simulink model "PubIfCommonEHRV2_MDL"  (R2020b)
settings: Solver=FixedStepAuto  StartTime=0.0  StopTime=Inf  RelTol=1e-3
PostLoadFcn:
  | if any(exist('dsrtsu_mdlpostloadfcn', 'file') ~= 0), dsrtsu_mdlpostloadfcn('Execute', bdroot); end
InitFcn:
  | , if any(exist('dsmpb_private', 'file') ~= 0), dsmpb_private('dsmpb_mdlclblib', 'Init', bdroot); end,
undefined symbols (not defined in the file): CAMERA_STATE_INITIAL, CAMERA_STATE_NORMAL, CURVATURE_UNKNOWN, DISTANCE_UNKONWN, DRIVING_ON_HIGHWAY_YES, EHR_CYCLE, FORWARD_LOOKING_DISTANCE_LIMIT, IFC_HUT_INTERFACE_NO_RESPONSE, IFC_HUT_INTERFACE_RESPONSE, MAP_DATA_VALID_VALID, MSG_TYPE_PROFILE_LONG, MSG_TYPE_PROFILE_SHORT, MSG_TYPE_SEGMENT, MSG_TYPE_STUB, OFFSET_INVALID, OFFSET_MAX, P_EHRV2_dCurvatureFar, P_EHRV2_dCurvatureMatrix, P_EHRV2_dSlopeFar, P_EHRV2_dSlopeMatrix, P_EHRV2_dVehForwardLooking, P_EHRV2_dVehRearLooking, P_EHRV2_tIFCHUTNoResponseOfForecastTreeReset, P_EHRV2_tIFCHUTNoResponseOfTimeout, P_EHRV2_tIFCHUTResponseTimeout, PROFILE_SHORT_NO_OTHER_VALUE, PROFILE_SHORT_TYPE_CURVATURE, PROFILE_SHORT_TYPE_SLOPE, REAR_LOOKING_DISTANCE_LIMIT, SLOPE_UNKNOWN, STUB_CMPLX_INSCT, STUB_FORM_OF_WAY_HIGH_RING_ROAD, STUB_FORM_OF_WAY_NORMAL_RING_ROAD
libraries: simulink x5
(part 1 of 4)
PreSaveFcn:
  | , if any(exist('dsmpb_private', 'file') ~= 0), dsmpb_private('dsmpb_mdlclblib', 'PreSave', bdroot); end,
CloseFcn:
  | , if any(exist('dsmpb_private', 'file') ~= 0), dsmpb_private('dsmpb_mdlclblib', 'Close', bdroot); end,
settings Model: DataDictionary=HWA_DDs.sldd  RTICANMMDATA=struct('GeneralSetupData',struct('modelroot','C:\Users\GW00133806\Desktop\ADAS_Store\Adas\EHR','generalsettings',struct('filesettings',struct('destfolder',struct('Name','RTICANMM_FILES','Check',1),'buildfolder',struct('Name','.','Check',1),'AbsDestfolder',struct('Name','C:\Users\GW00133806\Desktop\ADAS_Store\Adas\EHR\RTICANMM_FILES'),'AbsBuildfolder',struct('Name','C:\Users\GW00133806\Desktop\ADAS_Store\Adas\EHR'))),'options',struct('addpaths',1,'rmpaths',1,'addtrcexclusion',false,'cannavigator',struct('checkmonitoring',0),'show_usrtrc',0,'use_usrtrc',0),'advanced',struct('options',ones(1,100)),'MPSetup',{{}},'RTI',struct('Type','DSRT','Ver','4.2','Date','02-Nov-2019'),'modelname','PubIfCommonEHRV2_MDL','block','PubIfCommonEHRV2_MDL'))  DSRTSU_INTERNAL_RTIFPGA=150  Creator=GW00180895  LastModifiedBy=GW00133806
settings OptimizationCC: BlockReduction=off  ConditionallyExecuteInputs=off  OptimizeBlockIOStorage=off  BufferReuse=off  GlobalBufferReuse=off  ExpressionFolding=off  LocalBlockOutputs=off  OptimizeDataStoreBuffers=off  BusAssignmentInplaceUpdate=off
settings DebuggingCC: TasksWithSamePriorityMsg=none
settings HardwareCC: ProdBitPerPointer=32  ProdBitPerSizeT=32  ProdBitPerPtrDiffT=32  ProdLargestAtomicInteger=Integer  ProdWordSize=32  ProdHWDeviceType=Custom Processor->Custom
settings ModelReferenceCC: UpdateModelReferenceTargets=AssumeUpToDate  EnableParallelModelReferenceBuilds=on  ModelReferenceNumInstancesAllowed=Single
settings SFSimCC: MATLABDynamicMemAlloc=off
settings RTWCC: Description=dSPACE Run-Time Target (for VEOS on Windows and ConfigurationDesk)  SystemTargetFile=dsrt.tlc  GenCodeOnly=on  MakeCommand=make_dsrt  TemplateMakefile=dsrt_default_tmf  RTWVerbose=off
settings CodeAppCC: MaxIdLength=128
settings STFCustomTargetCC: TargetLangStandard=C99 (ISO)  ParMdlRefBuildCompliant=on  ConcurrentExecutionCompliant=off  CPPClassGenCompliant=off  GRTInterface=off  SystemTargetFile=dsrt.tlc
settings GRTTargetCC: CompOptLevelCompliant=off  ConcurrentExecutionCompliant=off  CombineOutputUpdateFcns=off  MatFileLogging=off  CPPClassGenCompliant=off  UseToolchainInfoCompliant=off

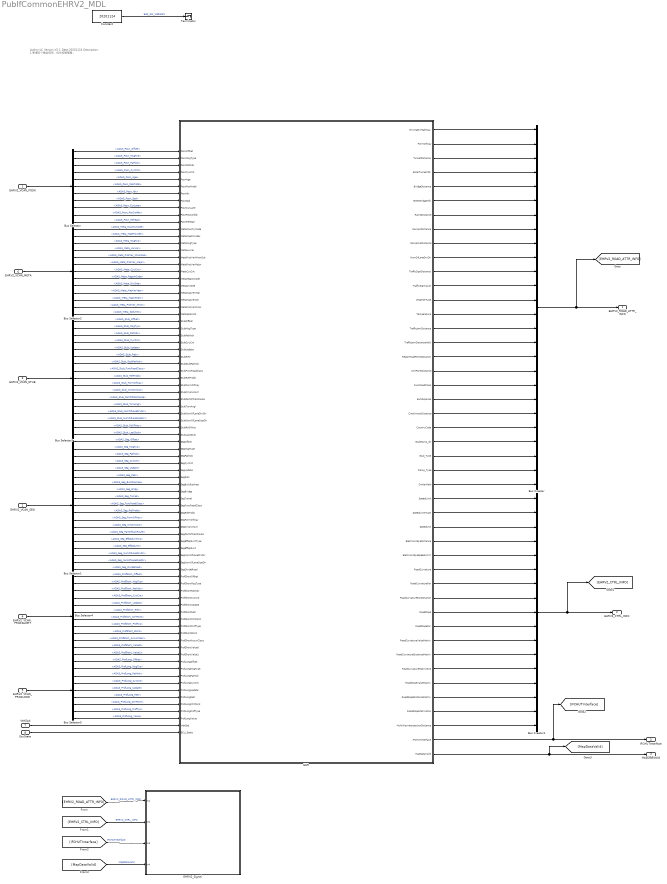
== system PubIfCommonEHRV2_MDL ==
  note: Author:LC
      | Version:V2.1
      | Data:20201124
      | Description:
      | 1.新增五个输出信号，优化控制策略；
  EHRV2_VCAN_POSN : Inport  OutDataTypeStr=Bus: EHRV2_VCAN_POSN_BUS  PortDimensions=1  BusOutputAsStruct=on
  EHRV2_VCAN_SEG : Inport  Port=2  OutDataTypeStr=Bus: EHRV2_VCAN_SEG_BUS  PortDimensions=1  BusOutputAsStruct=on
  EHRV2_VCAN_STUB : Inport  Port=3  OutDataTypeStr=Bus: EHRV2_VCAN_STUB_BUS  PortDimensions=1  BusOutputAsStruct=on
  EHRV2_VCAN_PROFSHORT : Inport  Port=4  OutDataTypeStr=Bus: EHRV2_VCAN_PROFSHORT_BUS  PortDimensions=1  BusOutputAsStruct=on
  EHRV2_VCAN_PROFLONG : Inport  Port=5  OutDataTypeStr=Bus: EHRV2_VCAN_PROFLONG_BUS  PortDimensions=1  BusOutputAsStruct=on
  EHRV2_VCAN_META : Inport  Port=6  OutDataTypeStr=Bus: EHRV2_VCAN_META_BUS  PortDimensions=1  BusOutputAsStruct=on
  VehSpd : Inport  Port=7  OutDataTypeStr=single  PortDimensions=1  BusOutputAsStruct=on
  EcuState : Inport  Port=8  OutDataTypeStr=uint8  PortDimensions=1  BusOutputAsStruct=on
  Bus Creator : BusCreator  Inputs=26
  Bus Creator1 : BusCreator  Inputs=17
  Bus Selector : BusSelector  OutputSignals=ADAS_Posn_Offset,ADAS_Posn_MsgTye,ADAS_Posn_Pathldx,ADAS_Posn_CycCnt,ADAS_Posn_Age,ADAS_Posn_PosProbb,ADAS_Posn_Idx,ADAS_Posn_Spd,ADAS_Posn_CurLane,ADAS_Posn_PosConfdc,ADAS_Posn_Rehead
  Bus Selector1 : BusSelector  OutputSignals=ADAS_Seg_Offset,ADAS_Seg_MsgTyp,ADAS_Seg_PathIdx,ADAS_Seg_CycCnt,ADAS_Seg_Update,ADAS_Seg_Retr,ADAS_Seg_BuildUpArea,ADAS_Seg_Brdg,ADAS_Seg_Tunnel,ADAS_Seg_FuncRoadClass,ADAS_Seg_RelProbb,ADAS_Seg_FormOfWay,ADAS_Seg_CmplxInsct,ADAS_Seg_PartOfCalcRoute,ADAS_Seg_EffSpdLmtTyp,ADAS_Seg_EffSpdLmt,ADAS_Seg_NumOfLaneDrvDir,ADAS_Seg_NumOfLaneOppDir,ADAS_Seg_DivideRoad
  Bus Selector2 : BusSelector  OutputSignals=ADAS_Meta_CountryCode,ADAS_Meta_MapProvider,ADAS_Meta_MsgTyp,ADAS_Meta_HwVer,ADAS_Meta_ProtVer_MinorSub,ADAS_Meta_ProtVer_Major,ADAS_Meta_CycCnt,ADAS_Meta_RegionCode,ADAS_Meta_DrvSide,ADAS_Meta_MapVerYear,ADAS_Meta_MapVerQtr,ADAS_Meta_ProtVer_Minor,ADAS_Meta_SpdUnits
  Bus Selector3 : BusSelector  OutputSignals=ADAS_Stub_Offset,ADAS_Stub_MsgTyp,ADAS_Stub_PathIdx,ADAS_Stub_CycCnt,ADAS_Stub_Update,ADAS_Stub_Retr,ADAS_Stub_StubPathIdx,ADAS_Stub_FuncRoadClass,ADAS_Stub_RelProbb,ADAS_Stub_FormOfWay,ADAS_Stub_CmplxInsct,ADAS_Stub_PartOfCalcRoute,ADAS_Stub_TurnAngl,ADAS_Stub_NumOfLaneDrvDir,ADAS_Stub_NumOfLaneOppDir,ADAS_Stub_RtOfWay,ADAS_Stub_LastStub
  Bus Selector4 : BusSelector  OutputSignals=ADAS_ProfShort_Offset,ADAS_ProfShort_MsgTyp,ADAS_ProfShort_PathIdx,ADAS_ProfShort_CycCnt,ADAS_ProfShort_Update,ADAS_ProfShort_Retr,ADAS_ProfShort_CtrlPoint,ADAS_ProfShort_ProfTyp,ADAS_ProfShort_Dist1,ADAS_ProfShort_AccurClass,ADAS_ProfShort_Value0,ADAS_ProfShort_Value1
  Bus Selector5 : BusSelector  OutputSignals=ADAS_ProfLong_Offset,ADAS_ProfLong_MsgTyp,ADAS_ProfLong_PathIdx,ADAS_ProfLong_CycCnt,ADAS_ProfLong_Update,ADAS_ProfLong_Retr,ADAS_ProfLong_CtrlPoint,ADAS_ProfLong_ProfTyp,ADAS_ProfLong_Value
  Constant : Constant  Value=20201124  OutDataTypeStr=uint32
  EHR : Subsystem
  EHRV2_Signal : Subsystem
  Terminator : Terminator
  EHRV2_ROAD_ATTR_INFO : Outport  OutDataTypeStr=Bus: EHRV2_ROAD_ATTR_INFO_BUS  PortDimensions=1  BusOutputAsStruct=on
  EHRV2_CTRL_INFO : Outport  Port=2  OutDataTypeStr=Bus: EHRV2_CTRL_INFO_BUS  PortDimensions=1  BusOutputAsStruct=on
  IFCHUTInterface : Outport  Port=3  OutDataTypeStr=uint8  PortDimensions=1  BusOutputAsStruct=on
  MapDataValid : Outport  Port=4  OutDataTypeStr=uint8  PortDimensions=1  BusOutputAsStruct=on
  wires:
  Bus Selector3/17 -> EHR/41(StubLastStub)  "<ADAS_Stub_LastStub>"
  EHR/25(Ramp_Type) -> Bus Creator/25
  Bus Selector3/16 -> EHR/40(StubRtOfWay)  "<ADAS_Stub_RtOfWay>"
  EHR/32(RoadCurvature) -> Bus Creator1/6
  Bus Selector1/11 -> EHR/52(SegRelProbb)  "<ADAS_Seg_RelProbb>"
  EHRV2_VCAN_SEG/1 -> Bus Selector1/1
  EHR/2(FormOfWay) -> Bus Creator/2
  Bus Selector/1 -> EHR/1(PosnOffset)  "<ADAS_Posn_Offset>"
  EHR/35(RoadSlope) -> Bus Creator1/9
  VehSpd/1 -> EHR/82(VehSpd)
  Bus Selector/4 -> EHR/4(PosnCycCnt)  "<ADAS_Posn_CycCnt>"
  EHRV2_VCAN_META/1 -> Bus Selector2/1
  Constant/1 -> Terminator/1  "EHR_SW_VERSION"
  EHR/11(TrafficSignDistance) -> Bus Creator/11
  EHR/36(RoadSlopeFar) -> Bus Creator1/10
  Bus Selector2/8 -> EHR/19(MetaRegionCode)  "<ADAS_Meta_RegionCode>"
  EHR/24(Stub_Type) -> Bus Creator/24
  EHR/12(TrafficSignValue) -> Bus Creator/12
  Bus Creator1/1 -> [EHRV2_CTRL_INFO], EHRV2_CTRL_INFO/1
  Bus Selector5/8 -> EHR/80(ProfLongProfType)  "<ADAS_ProfLong_ProfTyp>"
  Bus Selector/3 -> EHR/3(PosnPathIdx)  "<ADAS_Posn_Pathldx>"
  Bus Selector3/5 -> EHR/29(StubUpdate)  "<ADAS_Stub_Update>"
  EHR/23(StubRamp_dir) -> Bus Creator/23
  Bus Selector1/10 -> EHR/51(SegFuncRoadClass)  "<ADAS_Seg_FuncRoadClass>"
  Bus Selector4/4 -> EHR/64(ProfShortCycCnt)  "<ADAS_ProfShort_CycCnt>"
  EHR/43(MultiWayIntersectionDistance) -> Bus Creator1/17
  Bus Selector3/14 -> EHR/38(StubNumOfLaneDrvDir)  "<ADAS_Stub_NumOfLaneDrvDir>"
  Bus Selector2/7 -> EHR/18(MetaCycCnt)  "<ADAS_Meta_CycCnt>"
  EHRV2_VCAN_STUB/1 -> Bus Selector3/1
  EHRV2_VCAN_PROFSHORT/1 -> Bus Selector4/1
  EHR/9(RampOutDistance) -> Bus Creator/9
  EHR/39(RoadCurvatureMatrixSize) -> Bus Creator1/13
  EHRV2_VCAN_PROFLONG/1 -> Bus Selector5/1
  EHR/42(RoadSlopeMatrixSize) -> Bus Creator1/16
  EHR/15(TrafficJamDistance) -> Bus Creator/15
  EHR/29(SpeedUnit) -> Bus Creator1/3
  Bus Selector1/17 -> EHR/58(SegNumOfLaneDrvDir)  "<ADAS_Seg_NumOfLaneDrvDir>"
  Bus Selector4/7 -> EHR/67(ProfShortCtrlPoint)  "<ADAS_ProfShort_CtrlPoint>"
  Bus Selector4/10 -> EHR/70(ProfShortAccurClass)  "<ADAS_ProfShort_AccurClass>"
  Bus Selector3/10 -> EHR/34(StubFormOfWay)  "<ADAS_Stub_FormOfWay>"
  Bus Selector3/11 -> EHR/35(StubCmplxInsct)  "<ADAS_Stub_CmplxInsct>"
  Bus Selector2/6 -> EHR/17(MetaProtVerMajor)  "<ADAS_Meta_ProtVer_Major>"
  EHRV2_VCAN_POSN/1 -> Bus Selector/1
  EHR/41(RoadSlopeDistanceMatrix) -> Bus Creator1/15
  Bus Selector5/1 -> EHR/73(ProfLongOffset)  "<ADAS_ProfLong_Offset>"
  EHR/18(CtrlPointDistance) -> Bus Creator/18
  [IFCHUTInterface] -> EHRV2_Signal/3(In3)  "IFCHUTInterface"
  Bus Selector5/3 -> EHR/75(ProfLongPathIdx)  "<ADAS_ProfLong_PathIdx>"
  Bus Creator/1 -> [EHRV2_ROAD_ATTR_INFO], EHRV2_ROAD_ATTR_INFO/1
  EHR/45(MapDataValid) -> [MapDataValid], MapDataValid/1
  Bus Selector4/9 -> EHR/69(ProfShortDist1)  "<ADAS_ProfShort_Dist1>"
  Bus Selector/8 -> EHR/8(PosnSpd)  "<ADAS_Posn_Spd>"
  Bus Selector1/4 -> EHR/45(SegCycCnt)  "<ADAS_Seg_CycCnt>"
  Bus Selector/10 -> EHR/10(PosnPosConfdc)  "<ADAS_Posn_PosConfdc>"
  Bus Selector4/3 -> EHR/63(ProfShortPathIdx)  "<ADAS_ProfShort_PathIdx>"
  Bus Selector5/9 -> EHR/81(ProfLongValue)  "<ADAS_ProfLong_Value>"
  Bus Selector4/1 -> EHR/61(ProfShortOffset)  "<ADAS_ProfShort_Offset>"
  Bus Selector3/3 -> EHR/27(StubPathIdx)  "<ADAS_Stub_PathIdx>"
  Bus Selector5/4 -> EHR/76(ProfLongCycCnt)  "<ADAS_ProfLong_CycCnt>"
  EHR/17(RepairRoadPointDistance) -> Bus Creator/17
  Bus Selector3/13 -> EHR/37(StubTurnAngl)  "<ADAS_Stub_TurnAngl>"
  EHR/34(RoadCurvatureFarDistance) -> Bus Creator1/8
  EHR/8(RampInDistance) -> Bus Creator/8
  Bus Selector4/12 -> EHR/72(ProfShortValue1)  "<ADAS_ProfShort_Value1>"
  EHR/4(EnterTunnelInfo) -> Bus Creator/4
  Bus Selector2/9 -> EHR/20(MetaDrvSide)  "<ADAS_Meta_DrvSide>"
  EHR/26(OnNavPath) -> Bus Creator/26
  EHR/19(FuncRoadClass) -> Bus Creator/19
  Bus Selector5/7 -> EHR/79(ProfLongCtrlPoint)  "<ADAS_ProfLong_CtrlPoint>"
  Bus Selector1/5 -> EHR/46(SegUpdate)  "<ADAS_Seg_Update>"
  EHR/44(IFCHUTInterface) -> IFCHUTInterface/1, [IFCHUTInterface]
  Bus Selector2/11 -> EHR/22(MetaMapVerQtr)  "<ADAS_Meta_MapVerQtr>"
  Bus Selector3/7 -> EHR/31(StubStubPathIdx)  "<ADAS_Stub_StubPathIdx>"
  Bus Selector2/1 -> EHR/12(MetaCountryCode)  "<ADAS_Meta_CountryCode>"
  EHR/7(RampDistance) -> Bus Creator/7
  Bus Selector3/9 -> EHR/33(StubRelProbb)  "<ADAS_Stub_RelProbb>"
  Bus Selector1/3 -> EHR/44(SegPathIdx)  "<ADAS_Seg_PathIdx>"
  EcuState/1 -> EHR/83(ECU_State)
  Bus Selector1/7 -> EHR/48(SegBuildUpArea)  "<ADAS_Seg_BuildUpArea>"
  Bus Selector/6 -> EHR/6(PosnPosProbb)  "<ADAS_Posn_PosProbb>"
  Bus Selector3/8 -> EHR/32(StubFuncRoadClass)  "<ADAS_Stub_FuncRoadClass>"
  [EHRV2_CTRL_INFO] -> EHRV2_Signal/2(In2)  "EHRV2_CTRL_INFO"
  Bus Selector1/2 -> EHR/43(SegMsgType)  "<ADAS_Seg_MsgTyp>"
  Bus Selector2/3 -> EHR/14(MetaMsgType)  "<ADAS_Meta_MsgTyp>"
  Bus Selector2/5 -> EHR/16(MetaProtVerMinorSub)  "<ADAS_Meta_ProtVer_MinorSub>"
  Bus Selector/9 -> EHR/9(PosnCurLane)  "<ADAS_Posn_CurLane>"
  Bus Selector1/13 -> EHR/54(SegCmplxInsct)  "<ADAS_Seg_CmplxInsct>"
  Bus Selector3/15 -> EHR/39(StubNumOfLaneOppDir)  "<ADAS_Stub_NumOfLaneOppDir>"
  Bus Selector4/6 -> EHR/66(ProfShortRetr)  "<ADAS_ProfShort_Retr>"
  Bus Selector3/2 -> EHR/26(StubMsgType)  "<ADAS_Stub_MsgTyp>"
  Bus Selector1/19 -> EHR/60(SegDivideRoad)  "<ADAS_Seg_DivideRoad>"
  Bus Selector1/16 -> EHR/57(SegEffSpdLmt)  "<ADAS_Seg_EffSpdLmt>"
  Bus Selector4/2 -> EHR/62(ProfShortMsgType)  "<ADAS_ProfShort_MsgTyp>"
  EHR/37(RoadCurvatureValueMatrix) -> Bus Creator1/11
  Bus Selector2/10 -> EHR/21(MetaMapVerYear)  "<ADAS_Meta_MapVerYear>"
  Bus Selector2/2 -> EHR/13(MetaMapProvider)  "<ADAS_Meta_MapProvider>"
  Bus Selector/5 -> EHR/5(PosnAge)  "<ADAS_Posn_Age>"
  Bus Selector1/9 -> EHR/50(SegTunnel)  "<ADAS_Seg_Tunnel>"
  Bus Selector3/6 -> EHR/30(StubRetr)  "<ADAS_Stub_Retr>"
  Bus Selector1/8 -> EHR/49(SegBridge)  "<ADAS_Seg_Brdg>"
  Bus Selector/7 -> EHR/7(PosnIdx)  "<ADAS_Posn_Idx>"
  Bus Selector5/6 -> EHR/78(ProfLongRetr)  "<ADAS_ProfLong_Retr>"
  EHR/10(NumOfLaneDrvDir) -> Bus Creator/10
  Bus Selector5/5 -> EHR/77(ProfLongUpdate)  "<ADAS_ProfLong_Update>"
  Bus Selector2/13 -> EHR/24(MetaSpdUnits)  "<ADAS_Meta_SpdUnits>"
  EHR/30(ElectronicEyeDistance) -> Bus Creator1/4
  Bus Selector/11 -> EHR/11(PosnRehead)  "<ADAS_Posn_Rehead>"
  EHR/16(TrafficJamDistanceHold) -> Bus Creator/16
  EHR/31(ElectronicEyeSpeedLimit) -> Bus Creator1/5
  [EHRV2_ROAD_ATTR_INFO] -> EHRV2_Signal/1(In1)  "EHRV2_ROAD_ATTR_INFO"
  EHR/6(EnterBridgeInfo) -> Bus Creator/6
  Bus Selector4/8 -> EHR/68(ProfShortProfType)  "<ADAS_ProfShort_ProfTyp>"
  Bus Selector/2 -> EHR/2(PosnMsgType)  "<ADAS_Posn_MsgTye>"
  EHR/27(SpeedLimit) -> Bus Creator1/1
  EHR/22(CountryCode) -> Bus Creator/22
  Bus Selector3/12 -> EHR/36(StubPartOfCalcRoute)  "<ADAS_Stub_PartOfCalcRoute>"
  Bus Selector2/4 -> EHR/15(MetaHwVer)  "<ADAS_Meta_HwVer>"
  EHR/20(BuildUpArea) -> Bus Creator/20
  EHR/5(BridgeDistance) -> Bus Creator/5
  Bus Selector4/5 -> EHR/65(ProfShortUpdate)  "<ADAS_ProfShort_Update>"
  Bus Selector3/4 -> EHR/28(StubCycCnt)  "<ADAS_Stub_CycCnt>"
  Bus Selector1/14 -> EHR/55(SegPartOfCalcRoute)  "<ADAS_Seg_PartOfCalcRoute>"
  Bus Selector2/12 -> EHR/23(MetaProtVerMinor)  "<ADAS_Meta_ProtVer_Minor>"
  EHR/13(WeatherType) -> Bus Creator/13
  EHR/33(RoadCurvatureFar) -> Bus Creator1/7
  EHR/14(Temperature) -> Bus Creator/14
  Bus Selector4/11 -> EHR/71(ProfShortValue0)  "<ADAS_ProfShort_Value0>"
  Bus Selector1/18 -> EHR/59(SegNumOfLaneOppDir)  "<ADAS_Seg_NumOfLaneOppDir>"
  Bus Selector1/6 -> EHR/47(SegRetr)  "<ADAS_Seg_Retr>"
  EHR/3(TunnelDistance) -> Bus Creator/3
  Bus Selector1/12 -> EHR/53(SegFormOfWay)  "<ADAS_Seg_FormOfWay>"
  Bus Selector5/2 -> EHR/74(ProfLongMsgType)  "<ADAS_ProfLong_MsgTyp>"
  EHR/21(CmplxInsctDistance) -> Bus Creator/21
  [MapDataValid] -> EHRV2_Signal/4(In4)  "MapDataValid"
  Bus Selector1/15 -> EHR/56(SegEffSpdLmtType)  "<ADAS_Seg_EffSpdLmtTyp>"
  Bus Selector3/1 -> EHR/25(StubOffset)  "<ADAS_Stub_Offset>"
  Bus Selector1/1 -> EHR/42(SegOffset)  "<ADAS_Seg_Offset>"
  EHR/28(SpeedLimitType) -> Bus Creator1/2
  EHR/1(DrivingOnHighWay) -> Bus Creator/1
  EHR/40(RoadSlopeValueMatrix) -> Bus Creator1/14
  EHR/38(RoadCurvatureDistanceMatrix) -> Bus Creator1/12

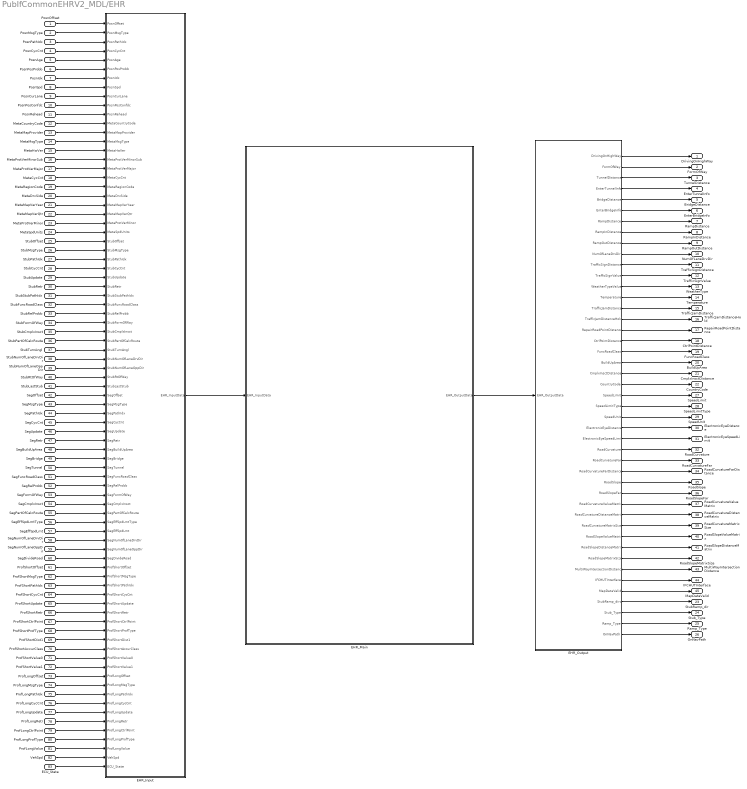
== system PubIfCommonEHRV2_MDL/EHR ==
  PosnOffset : Inport  OutDataTypeStr=uint16  PortDimensions=1
  PosnMsgType : Inport  Port=2  OutDataTypeStr=uint8  PortDimensions=1
  PosnPathIdx : Inport  Port=3  OutDataTypeStr=uint8  PortDimensions=1
  PosnCycCnt : Inport  Port=4  OutDataTypeStr=uint8  PortDimensions=1
  PosnAge : Inport  Port=5  OutDataTypeStr=uint16  PortDimensions=1
  PosnPosProbb : Inport  Port=6  OutDataTypeStr=single  PortDimensions=1
  PosnIdx : Inport  Port=7  OutDataTypeStr=uint8  PortDimensions=1
  PosnSpd : Inport  Port=8  OutDataTypeStr=single  PortDimensions=1
  PosnCurLane : Inport  Port=9  OutDataTypeStr=uint8  PortDimensions=1
  PosnPosConfdc : Inport  Port=10  OutDataTypeStr=uint8  PortDimensions=1
  PosnRehead : Inport  Port=11  OutDataTypeStr=single  PortDimensions=1
  MetaCountryCode : Inport  Port=12  OutDataTypeStr=uint16  PortDimensions=1
  MetaMapProvider : Inport  Port=13  OutDataTypeStr=uint8  PortDimensions=1
  MetaMsgType : Inport  Port=14  OutDataTypeStr=uint8  PortDimensions=1
  MetaHwVer : Inport  Port=15  OutDataTypeStr=uint16  PortDimensions=1
  MetaProtVerMinorSub : Inport  Port=16  OutDataTypeStr=uint8  PortDimensions=1
  MetaProtVerMajor : Inport  Port=17  OutDataTypeStr=uint8  PortDimensions=1
  MetaCycCnt : Inport  Port=18  OutDataTypeStr=uint8  PortDimensions=1
  MetaRegionCode : Inport  Port=19  OutDataTypeStr=uint16  PortDimensions=1
  MetaDrvSide : Inport  Port=20  OutDataTypeStr=boolean  PortDimensions=1
  MetaMapVerYear : Inport  Port=21  OutDataTypeStr=uint8  PortDimensions=1
  MetaMapVerQtr : Inport  Port=22  OutDataTypeStr=uint8  PortDimensions=1
  MetaProtVerMinor : Inport  Port=23  OutDataTypeStr=uint8  PortDimensions=1
  MetaSpdUnits : Inport  Port=24  OutDataTypeStr=boolean  PortDimensions=1
  StubOffset : Inport  Port=25  OutDataTypeStr=uint16  PortDimensions=1
  StubMsgType : Inport  Port=26  OutDataTypeStr=uint8  PortDimensions=1
  StubPathIdx : Inport  Port=27  OutDataTypeStr=uint8  PortDimensions=1
  StubCycCnt : Inport  Port=28  OutDataTypeStr=uint8  PortDimensions=1
  StubUpdate : Inport  Port=29  OutDataTypeStr=boolean  PortDimensions=1
  StubRetr : Inport  Port=30  OutDataTypeStr=boolean  PortDimensions=1
  StubStubPathIdx : Inport  Port=31  OutDataTypeStr=uint8  PortDimensions=1
  StubFuncRoadClass : Inport  Port=32  OutDataTypeStr=uint8  PortDimensions=1
  StubRelProbb : Inport  Port=33  OutDataTypeStr=single  PortDimensions=1
  StubFormOfWay : Inport  Port=34  OutDataTypeStr=uint8  PortDimensions=1
  StubCmplxInsct : Inport  Port=35  OutDataTypeStr=uint8  PortDimensions=1
  StubPartOfCalcRoute : Inport  Port=36  OutDataTypeStr=uint8  PortDimensions=1
  StubTurnAngl : Inport  Port=37  OutDataTypeStr=single  PortDimensions=1
  StubNumOfLaneDrvDir : Inport  Port=38  OutDataTypeStr=uint8  PortDimensions=1
  StubNumOfLaneOppDir : Inport  Port=39  OutDataTypeStr=uint8  PortDimensions=1
  StubRtOfWay : Inport  Port=40  OutDataTypeStr=uint8  PortDimensions=1
  StubLastStub : Inport  Port=41  OutDataTypeStr=boolean  PortDimensions=1
  SegOffset : Inport  Port=42  OutDataTypeStr=uint16  PortDimensions=1
  SegMsgType : Inport  Port=43  OutDataTypeStr=uint8  PortDimensions=1
  SegPathIdx : Inport  Port=44  OutDataTypeStr=uint8  PortDimensions=1
  SegCycCnt : Inport  Port=45  OutDataTypeStr=uint8  PortDimensions=1
  SegUpdate : Inport  Port=46  OutDataTypeStr=boolean  PortDimensions=1
  SegRetr : Inport  Port=47  OutDataTypeStr=boolean  PortDimensions=1
  SegBuildUpArea : Inport  Port=48  OutDataTypeStr=uint8  PortDimensions=1
  SegBridge : Inport  Port=49  OutDataTypeStr=uint8  PortDimensions=1
  SegTunnel : Inport  Port=50  OutDataTypeStr=uint8  PortDimensions=1
  SegFuncRoadClass : Inport  Port=51  OutDataTypeStr=uint8  PortDimensions=1
  SegRelProbb : Inport  Port=52  OutDataTypeStr=single  PortDimensions=1
  SegFormOfWay : Inport  Port=53  OutDataTypeStr=uint8  PortDimensions=1
  SegCmplxInsct : Inport  Port=54  OutDataTypeStr=uint8  PortDimensions=1
  SegPartOfCalcRoute : Inport  Port=55  OutDataTypeStr=uint8  PortDimensions=1
  SegEffSpdLmtType : Inport  Port=56  OutDataTypeStr=uint8  PortDimensions=1
  SegEffSpdLmt : Inport  Port=57  OutDataTypeStr=uint8  PortDimensions=1
  SegNumOfLaneDrvDir : Inport  Port=58  OutDataTypeStr=uint8  PortDimensions=1
  SegNumOfLaneOppDir : Inport  Port=59  OutDataTypeStr=uint8  PortDimensions=1
  SegDivideRoad : Inport  Port=60  OutDataTypeStr=uint8  PortDimensions=1
  ProfShortOffset : Inport  Port=61  OutDataTypeStr=uint16  PortDimensions=1
  ProfShortMsgType : Inport  Port=62  OutDataTypeStr=uint8  PortDimensions=1
  ProfShortPathIdx : Inport  Port=63  OutDataTypeStr=uint8  PortDimensions=1
  ProfShortCycCnt : Inport  Port=64  OutDataTypeStr=uint8  PortDimensions=1
  ProfShortUpdate : Inport  Port=65  OutDataTypeStr=boolean  PortDimensions=1
  ProfShortRetr : Inport  Port=66  OutDataTypeStr=boolean  PortDimensions=1
  ProfShortCtrlPoint : Inport  Port=67  OutDataTypeStr=boolean  PortDimensions=1
  ProfShortProfType : Inport  Port=68  OutDataTypeStr=uint8  PortDimensions=1
  ProfShortDist1 : Inport  Port=69  OutDataTypeStr=uint16  PortDimensions=1
  ProfShortAccurClass : Inport  Port=70  OutDataTypeStr=uint8  PortDimensions=1
  ProfShortValue0 : Inport  Port=71  OutDataTypeStr=uint16  PortDimensions=1
  ProfShortValue1 : Inport  Port=72  OutDataTypeStr=uint16  PortDimensions=1
  ProfLongOffset : Inport  Port=73  OutDataTypeStr=uint16  PortDimensions=1
  ProfLongMsgType : Inport  Port=74  OutDataTypeStr=uint8  PortDimensions=1
  ProfLongPathIdx : Inport  Port=75  OutDataTypeStr=uint8  PortDimensions=1
  ProfLongCycCnt : Inport  Port=76  OutDataTypeStr=uint8  PortDimensions=1
  ProfLongUpdate : Inport  Port=77  OutDataTypeStr=boolean  PortDimensions=1
  ProfLongRetr : Inport  Port=78  OutDataTypeStr=boolean  PortDimensions=1
  ProfLongCtrlPoint : Inport  Port=79  OutDataTypeStr=boolean  PortDimensions=1
  ProfLongProfType : Inport  Port=80  OutDataTypeStr=uint8  PortDimensions=1
  ProfLongValue : Inport  Port=81  OutDataTypeStr=uint32  PortDimensions=1
  VehSpd : Inport  Port=82  OutDataTypeStr=single  PortDimensions=1
  ECU_State : Inport  Port=83  OutDataTypeStr=uint8  PortDimensions=1
  EHR_Input : Subsystem
  EHR_Main : Subsystem
  EHR_Output : Subsystem
  DrivingOnHighWay : Outport  OutDataTypeStr=uint8  PortDimensions=1
  FormOfWay : Outport  Port=2  OutDataTypeStr=uint8  PortDimensions=1
  TunnelDistance : Outport  Port=3  OutDataTypeStr=uint16  PortDimensions=1
  EnterTunnelInfo : Outport  Port=4  OutDataTypeStr=uint8  PortDimensions=1
  BridgeDistance : Outport  Port=5  OutDataTypeStr=uint16  PortDimensions=1
  EnterBridgeInfo : Outport  Port=6  OutDataTypeStr=uint8  PortDimensions=1
  RampDistance : Outport  Port=7  OutDataTypeStr=uint16  PortDimensions=1
  RampInDistance : Outport  Port=8  OutDataTypeStr=uint16  PortDimensions=1
  RampOutDistance : Outport  Port=9  OutDataTypeStr=uint16  PortDimensions=1
  NumOfLaneDrvDir : Outport  Port=10  OutDataTypeStr=uint8  PortDimensions=1
  TrafficSignDistance : Outport  Port=11  OutDataTypeStr=uint16  PortDimensions=1
  TrafficSignValue : Outport  Port=12  OutDataTypeStr=uint8  PortDimensions=1
  WeatherType : Outport  Port=13  OutDataTypeStr=uint8  PortDimensions=1
  Temperature : Outport  Port=14  OutDataTypeStr=int8  PortDimensions=1
  TrafficJamDistance : Outport  Port=15  OutDataTypeStr=uint16  PortDimensions=1
  TrafficJamDistanceHold : Outport  Port=16  OutDataTypeStr=uint16  PortDimensions=1
  RepairRoadPointDistance : Outport  Port=17  OutDataTypeStr=uint16  PortDimensions=1
  CtrlPointDistance : Outport  Port=18  OutDataTypeStr=uint16  PortDimensions=1
  FuncRoadClass : Outport  Port=19  OutDataTypeStr=uint8  PortDimensions=1
  BuildUpArea : Outport  Port=20  OutDataTypeStr=uint8  PortDimensions=1
  CmplxInsctDistance : Outport  Port=21  OutDataTypeStr=uint16  PortDimensions=1
  CountryCode : Outport  Port=22  OutDataTypeStr=uint16  PortDimensions=1
  StubRamp_dir : Outport  Port=23  OutDataTypeStr=uint8  PortDimensions=1
  Stub_Type : Outport  Port=24  OutDataTypeStr=uint8  PortDimensions=1
  Ramp_Type : Outport  Port=25  OutDataTypeStr=uint8  PortDimensions=1
  OnNavPath : Outport  Port=26  OutDataTypeStr=uint8  PortDimensions=1
  SpeedLimit : Outport  Port=27  OutDataTypeStr=uint8  PortDimensions=1
  SpeedLimitType : Outport  Port=28  OutDataTypeStr=uint8  PortDimensions=1
  SpeedUnit : Outport  Port=29  OutDataTypeStr=uint8  PortDimensions=1
  ElectronicEyeDistance : Outport  Port=30  OutDataTypeStr=uint16  PortDimensions=1
  ElectronicEyeSpeedLimit : Outport  Port=31  OutDataTypeStr=uint8  PortDimensions=1
  RoadCurvature : Outport  Port=32  OutDataTypeStr=single  PortDimensions=1
  RoadCurvatureFar : Outport  Port=33  OutDataTypeStr=single  PortDimensions=1
  RoadCurvatureFarDistance : Outport  Port=34  OutDataTypeStr=uint16  PortDimensions=1
  RoadSlope : Outport  Port=35  OutDataTypeStr=single  PortDimensions=1
  RoadSlopeFar : Outport  Port=36  OutDataTypeStr=single  PortDimensions=1
  RoadCurvatureValueMatrix : Outport  Port=37  OutDataTypeStr=single  PortDimensions=10
  RoadCurvatureDistanceMatrix : Outport  Port=38  OutDataTypeStr=single  PortDimensions=10
  RoadCurvatureMatrixSize : Outport  Port=39  OutDataTypeStr=uint8  PortDimensions=1
  RoadSlopeValueMatrix : Outport  Port=40  OutDataTypeStr=single  PortDimensions=10
  RoadSlopeDistanceMatrix : Outport  Port=41  OutDataTypeStr=single  PortDimensions=10
  RoadSlopeMatrixSize : Outport  Port=42  OutDataTypeStr=uint8  PortDimensions=1
  MultiWayIntersectionDistance : Outport  Port=43  OutDataTypeStr=uint16  PortDimensions=1
  IFCHUTInterface : Outport  Port=44  OutDataTypeStr=uint8  PortDimensions=1
  MapDataValid : Outport  Port=45  OutDataTypeStr=uint8  PortDimensions=1
  wires:
  PosnOffset/1 -> EHR_Input/1(PosnOffset)
  PosnMsgType/1 -> EHR_Input/2(PosnMsgType)
  PosnPathIdx/1 -> EHR_Input/3(PosnPathIdx)
  PosnCycCnt/1 -> EHR_Input/4(PosnCycCnt)
  PosnAge/1 -> EHR_Input/5(PosnAge)
  PosnPosProbb/1 -> EHR_Input/6(PosnPosProbb)
  PosnIdx/1 -> EHR_Input/7(PosnIdx)
  PosnSpd/1 -> EHR_Input/8(PosnSpd)
  PosnCurLane/1 -> EHR_Input/9(PosnCurLane)
  PosnPosConfdc/1 -> EHR_Input/10(PosnPosConfdc)
  PosnRehead/1 -> EHR_Input/11(PosnRehead)
  MetaCountryCode/1 -> EHR_Input/12(MetaCountryCode)
  MetaMapProvider/1 -> EHR_Input/13(MetaMapProvider)
  MetaMsgType/1 -> EHR_Input/14(MetaMsgType)
  MetaHwVer/1 -> EHR_Input/15(MetaHwVer)
  MetaProtVerMinorSub/1 -> EHR_Input/16(MetaProtVerMinorSub)
  MetaProtVerMajor/1 -> EHR_Input/17(MetaProtVerMajor)
  MetaCycCnt/1 -> EHR_Input/18(MetaCycCnt)
  MetaRegionCode/1 -> EHR_Input/19(MetaRegionCode)
  MetaDrvSide/1 -> EHR_Input/20(MetaDrvSide)
  MetaMapVerYear/1 -> EHR_Input/21(MetaMapVerYear)
  MetaMapVerQtr/1 -> EHR_Input/22(MetaMapVerQtr)
  MetaProtVerMinor/1 -> EHR_Input/23(MetaProtVerMinor)
  MetaSpdUnits/1 -> EHR_Input/24(MetaSpdUnits)
  StubOffset/1 -> EHR_Input/25(StubOffset)
  StubMsgType/1 -> EHR_Input/26(StubMsgType)
  StubPathIdx/1 -> EHR_Input/27(StubPathIdx)
  StubCycCnt/1 -> EHR_Input/28(StubCycCnt)
  StubUpdate/1 -> EHR_Input/29(StubUpdate)
  StubRetr/1 -> EHR_Input/30(StubRetr)
  StubStubPathIdx/1 -> EHR_Input/31(StubStubPathIdx)
  StubFuncRoadClass/1 -> EHR_Input/32(StubFuncRoadClass)
  StubRelProbb/1 -> EHR_Input/33(StubRelProbb)
  StubFormOfWay/1 -> EHR_Input/34(StubFormOfWay)
  StubCmplxInsct/1 -> EHR_Input/35(StubCmplxInsct)
  StubPartOfCalcRoute/1 -> EHR_Input/36(StubPartOfCalcRoute)
  StubTurnAngl/1 -> EHR_Input/37(StubTurnAngl)
  StubNumOfLaneDrvDir/1 -> EHR_Input/38(StubNumOfLaneDrvDir)
  StubNumOfLaneOppDir/1 -> EHR_Input/39(StubNumOfLaneOppDir)
  StubRtOfWay/1 -> EHR_Input/40(StubRtOfWay)
  StubLastStub/1 -> EHR_Input/41(StubLastStub)
  SegOffset/1 -> EHR_Input/42(SegOffset)
  SegMsgType/1 -> EHR_Input/43(SegMsgType)
  SegPathIdx/1 -> EHR_Input/44(SegPathIdx)
  SegCycCnt/1 -> EHR_Input/45(SegCycCnt)
  SegUpdate/1 -> EHR_Input/46(SegUpdate)
  SegRetr/1 -> EHR_Input/47(SegRetr)
  SegBuildUpArea/1 -> EHR_Input/48(SegBuildUpArea)
  SegBridge/1 -> EHR_Input/49(SegBridge)
  SegTunnel/1 -> EHR_Input/50(SegTunnel)
  SegFuncRoadClass/1 -> EHR_Input/51(SegFuncRoadClass)
  SegRelProbb/1 -> EHR_Input/52(SegRelProbb)
  SegFormOfWay/1 -> EHR_Input/53(SegFormOfWay)
  SegCmplxInsct/1 -> EHR_Input/54(SegCmplxInsct)
  SegPartOfCalcRoute/1 -> EHR_Input/55(SegPartOfCalcRoute)
  SegEffSpdLmtType/1 -> EHR_Input/56(SegEffSpdLmtType)
  SegEffSpdLmt/1 -> EHR_Input/57(SegEffSpdLmt)
  SegNumOfLaneDrvDir/1 -> EHR_Input/58(SegNumOfLaneDrvDir)
  SegNumOfLaneOppDir/1 -> EHR_Input/59(SegNumOfLaneOppDir)
  SegDivideRoad/1 -> EHR_Input/60(SegDivideRoad)
  ProfShortOffset/1 -> EHR_Input/61(ProfShortOffset)
  ProfShortMsgType/1 -> EHR_Input/62(ProfShortMsgType)
  ProfShortPathIdx/1 -> EHR_Input/63(ProfShortPathIdx)
  ProfShortCycCnt/1 -> EHR_Input/64(ProfShortCycCnt)
  ProfShortUpdate/1 -> EHR_Input/65(ProfShortUpdate)
  ProfShortRetr/1 -> EHR_Input/66(ProfShortRetr)
  ProfShortCtrlPoint/1 -> EHR_Input/67(ProfShortCtrlPoint)
  ProfShortProfType/1 -> EHR_Input/68(ProfShortProfType)
  ProfShortDist1/1 -> EHR_Input/69(ProfShortDist1)
  ProfShortAccurClass/1 -> EHR_Input/70(ProfShortAccurClass)
  ProfShortValue0/1 -> EHR_Input/71(ProfShortValue0)
  ProfShortValue1/1 -> EHR_Input/72(ProfShortValue1)
  ProfLongOffset/1 -> EHR_Input/73(ProfLongOffset)
  ProfLongMsgType/1 -> EHR_Input/74(ProfLongMsgType)
  ProfLongPathIdx/1 -> EHR_Input/75(ProfLongPathIdx)
  ProfLongCycCnt/1 -> EHR_Input/76(ProfLongCycCnt)
  ProfLongUpdate/1 -> EHR_Input/77(ProfLongUpdate)
  ProfLongRetr/1 -> EHR_Input/78(ProfLongRetr)
  ProfLongCtrlPoint/1 -> EHR_Input/79(ProfLongCtrlPoint)
  ProfLongProfType/1 -> EHR_Input/80(ProfLongProfType)
  ProfLongValue/1 -> EHR_Input/81(ProfLongValue)
  VehSpd/1 -> EHR_Input/82(VehSpd)
  ECU_State/1 -> EHR_Input/83(ECU_State)
  EHR_Output/1(DrivingOnHighWay) -> DrivingOnHighWay/1
  EHR_Output/10(NumOfLaneDrvDir) -> NumOfLaneDrvDir/1
  EHR_Output/2(FormOfWay) -> FormOfWay/1
  EHR_Output/5(BridgeDistance) -> BridgeDistance/1
  EHR_Output/4(EnterTunnelInfo) -> EnterTunnelInfo/1
  EHR_Output/3(TunnelDistance) -> TunnelDistance/1
  EHR_Output/7(RampDistance) -> RampDistance/1
  EHR_Output/6(EnterBridgeInfo) -> EnterBridgeInfo/1
  EHR_Input/1(EHR_InputData) -> EHR_Main/1(EHR_InputData)
  EHR_Main/1(EHR_OutputData) -> EHR_Output/1(EHR_OutputData)
  EHR_Output/8(RampInDistance) -> RampInDistance/1
  EHR_Output/9(RampOutDistance) -> RampOutDistance/1
  EHR_Output/11(TrafficSignDistance) -> TrafficSignDistance/1
  EHR_Output/12(TrafficSignValue) -> TrafficSignValue/1
  EHR_Output/13(WeatherTypeValue) -> WeatherType/1
  EHR_Output/14(Temperature) -> Temperature/1
  EHR_Output/15(TrafficJamDistance) -> TrafficJamDistance/1
  EHR_Output/16(TrafficJamDistanceHold) -> TrafficJamDistanceHold/1
  EHR_Output/17(RepairRoadPointDistance) -> RepairRoadPointDistance/1
  EHR_Output/18(CtrlPointDistance) -> CtrlPointDistance/1
  EHR_Output/19(FuncRoadClass) -> FuncRoadClass/1
  EHR_Output/20(BuildUpArea) -> BuildUpArea/1
  EHR_Output/21(CmplxInsctDistance) -> CmplxInsctDistance/1
  EHR_Output/22(CountryCode) -> CountryCode/1
  EHR_Output/23(SpeedLimit) -> SpeedLimit/1
  EHR_Output/24(SpeedLimitType) -> SpeedLimitType/1
  EHR_Output/25(SpeedUnit) -> SpeedUnit/1
  EHR_Output/26(ElectronicEyeDistance) -> ElectronicEyeDistance/1
  EHR_Output/27(ElectronicEyeSpeedLimit) -> ElectronicEyeSpeedLimit/1
  EHR_Output/28(RoadCurvature) -> RoadCurvature/1
  EHR_Output/29(RoadCurvatureFar) -> RoadCurvatureFar/1
  EHR_Output/30(RoadCurvatureFarDistance) -> RoadCurvatureFarDistance/1
  EHR_Output/31(RoadSlope) -> RoadSlope/1
  EHR_Output/32(RoadSlopeFar) -> RoadSlopeFar/1
  EHR_Output/33(RoadCurvatureValueMatrix) -> RoadCurvatureValueMatrix/1
  EHR_Output/34(RoadCurvatureDistanceMatrix) -> RoadCurvatureDistanceMatrix/1
  EHR_Output/35(RoadCurvatureMatrixSize) -> RoadCurvatureMatrixSize/1
  EHR_Output/36(RoadSlopeValueMatrix) -> RoadSlopeValueMatrix/1
  EHR_Output/37(RoadSlopeDistanceMatrix) -> RoadSlopeDistanceMatrix/1
  EHR_Output/38(RoadSlopeMatrixSize) -> RoadSlopeMatrixSize/1
  EHR_Output/40(IFCHUTInterface) -> IFCHUTInterface/1
  EHR_Output/41(MapDataValid) -> MapDataValid/1
  EHR_Output/39(MultiWayIntersectionDistance) -> MultiWayIntersectionDistance/1
  EHR_Output/42(StubRamp_dirc) -> StubRamp_dir/1
  EHR_Output/43(Stub_Type) -> Stub_Type/1
  EHR_Output/44(Ramp_Type) -> Ramp_Type/1
  EHR_Output/45(OnNavPath) -> OnNavPath/1

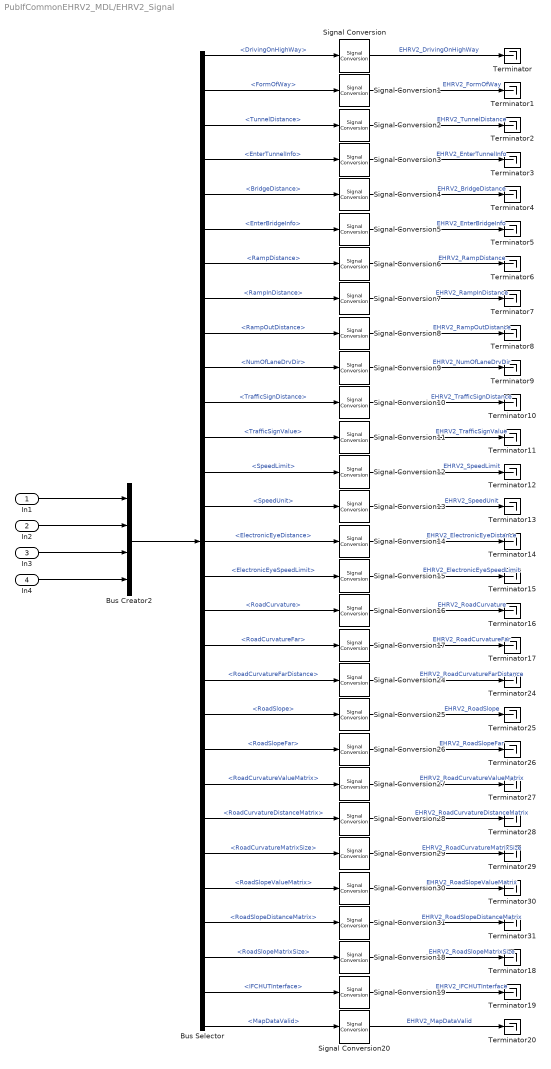
== system PubIfCommonEHRV2_MDL/EHRV2_Signal ==
  In1 : Inport
  In2 : Inport  Port=2
  In3 : Inport  Port=3
  In4 : Inport  Port=4
  Bus Creator2 : BusCreator  Inputs=4
  Bus Selector : BusSelector  OutputSignals=EHRV2_ROAD_ATTR_INFO.DrivingOnHighWay,EHRV2_ROAD_ATTR_INFO.FormOfWay,EHRV2_ROAD_ATTR_INFO.TunnelDistance,EHRV2_ROAD_ATTR_INFO.EnterTunnelInfo,EHRV2_ROAD_ATTR_INFO.BridgeDistance,EHRV2_ROAD_ATTR_INFO.EnterBridgeInfo,EHRV2_ROAD_ATTR_INFO.RampDistance,EHRV2_ROAD_ATTR_INFO.RampInDistance,EHRV2_ROAD_ATTR_INFO.RampOutDistance,EHRV2_ROAD_ATTR_INFO.NumOfLaneDrvDir,EHRV2_ROAD_ATTR_INFO.TrafficSignDistance,EHRV2_ROAD_ATTR_INFO.TrafficSignValue,EHRV2_CTRL_INFO.SpeedLimit,EHRV2_CTRL_INFO.SpeedUnit,EHRV2_CTRL_INFO.ElectronicEyeDistance,EHRV2_CTRL_INFO.ElectronicEyeSpeedLimit,EHRV2_CTRL_INFO.RoadCurvature,EHRV2_CTRL_INFO.RoadCurvatureFar,EHRV2_CTRL_INFO.RoadCurvatureFarDistance,EHRV2_CTRL_INFO.RoadSlope,EHRV2_CTRL_INFO.RoadSlopeFar,EHRV2_CTRL_INFO.RoadCurvatureValueMatrix,EHRV2_CTRL_INFO.RoadCurvatureDistanceMatrix,EHRV2_CTRL_INFO.RoadCurvatureMatrixSize,EHRV2_CTRL_INFO.RoadSlopeValueMatrix,EHRV2_CTRL_INFO.RoadSlopeDistanceMatrix,EHRV2_CTRL_INFO.RoadSlopeMatrixSize,IFCHUTInterface,MapDataValid
  Signal Conversion{,1..20,24..31} (29 alike) : SignalConversion  OverrideOpt=off
  Terminator{,1..20,24..31} (29 alike) : Terminator
  wires:
  In2/1 -> Bus Creator2/2
  Bus Creator2/1 -> Bus Selector/1
  In1/1 -> Bus Creator2/1
  Bus Selector/1 -> Signal Conversion/1  "<DrivingOnHighWay>"
  Signal Conversion/1 -> Terminator/1  "EHRV2_DrivingOnHighWay"
  Signal Conversion1/1 -> Terminator1/1  "EHRV2_FormOfWay"
  Bus Selector/2 -> Signal Conversion1/1  "<FormOfWay>"
  Bus Selector/4 -> Signal Conversion3/1  "<EnterTunnelInfo>"
  Signal Conversion3/1 -> Terminator3/1  "EHRV2_EnterTunnelInfo"
  Signal Conversion2/1 -> Terminator2/1  "EHRV2_TunnelDistance"
  Bus Selector/3 -> Signal Conversion2/1  "<TunnelDistance>"
  Bus Selector/7 -> Signal Conversion6/1  "<RampDistance>"
  Signal Conversion6/1 -> Terminator6/1  "EHRV2_RampDistance"
  Signal Conversion7/1 -> Terminator7/1  "EHRV2_RampInDistance"
  Bus Selector/8 -> Signal Conversion7/1  "<RampInDistance>"
  Bus Selector/6 -> Signal Conversion5/1  "<EnterBridgeInfo>"
  Signal Conversion5/1 -> Terminator5/1  "EHRV2_EnterBridgeInfo"
  Signal Conversion4/1 -> Terminator4/1  "EHRV2_BridgeDistance"
  Bus Selector/5 -> Signal Conversion4/1  "<BridgeDistance>"
  Bus Selector/13 -> Signal Conversion12/1  "<SpeedLimit>"
  Signal Conversion12/1 -> Terminator12/1  "EHRV2_SpeedLimit"
  Signal Conversion13/1 -> Terminator13/1  "EHRV2_SpeedUnit"
  Bus Selector/14 -> Signal Conversion13/1  "<SpeedUnit>"
  Bus Selector/16 -> Signal Conversion15/1  "<ElectronicEyeSpeedLimit>"
  Signal Conversion15/1 -> Terminator15/1  "EHRV2_ElectronicEyeSpeedLimit"
  Signal Conversion14/1 -> Terminator14/1  "EHRV2_ElectronicEyeDistance"
  Bus Selector/15 -> Signal Conversion14/1  "<ElectronicEyeDistance>"
  Bus Selector/11 -> Signal Conversion10/1  "<TrafficSignDistance>"
  Signal Conversion10/1 -> Terminator10/1  "EHRV2_TrafficSignDistance"
  Signal Conversion11/1 -> Terminator11/1  "EHRV2_TrafficSignValue"
  Bus Selector/12 -> Signal Conversion11/1  "<TrafficSignValue>"
  Bus Selector/10 -> Signal Conversion9/1  "<NumOfLaneDrvDir>"
  Signal Conversion9/1 -> Terminator9/1  "EHRV2_NumOfLaneDrvDir"
  Signal Conversion8/1 -> Terminator8/1  "EHRV2_RampOutDistance"
  Bus Selector/9 -> Signal Conversion8/1  "<RampOutDistance>"
  Bus Selector/25 -> Signal Conversion30/1  "<RoadSlopeValueMatrix>"
  Signal Conversion30/1 -> Terminator30/1  "EHRV2_RoadSlopeValueMatrix"
  Signal Conversion31/1 -> Terminator31/1  "EHRV2_RoadSlopeDistanceMatrix"
  Bus Selector/26 -> Signal Conversion31/1  "<RoadSlopeDistanceMatrix>"
  Signal Conversion18/1 -> Terminator18/1  "EHRV2_RoadSlopeMatrixSize"
  Bus Selector/27 -> Signal Conversion18/1  "<RoadSlopeMatrixSize>"
  Bus Selector/21 -> Signal Conversion26/1  "<RoadSlopeFar>"
  Signal Conversion26/1 -> Terminator26/1  "EHRV2_RoadSlopeFar"
  Signal Conversion27/1 -> Terminator27/1  "EHRV2_RoadCurvatureValueMatrix"
  Bus Selector/22 -> Signal Conversion27/1  "<RoadCurvatureValueMatrix>"
  Bus Selector/24 -> Signal Conversion29/1  "<RoadCurvatureMatrixSize>"
  Signal Conversion29/1 -> Terminator29/1  "EHRV2_RoadCurvatureMatrixSize"
  Signal Conversion28/1 -> Terminator28/1  "EHRV2_RoadCurvatureDistanceMatrix"
  Bus Selector/23 -> Signal Conversion28/1  "<RoadCurvatureDistanceMatrix>"
  Bus Selector/19 -> Signal Conversion24/1  "<RoadCurvatureFarDistance>"
  Signal Conversion24/1 -> Terminator24/1  "EHRV2_RoadCurvatureFarDistance"
  Signal Conversion25/1 -> Terminator25/1  "EHRV2_RoadSlope"
  Bus Selector/20 -> Signal Conversion25/1  "<RoadSlope>"
  Bus Selector/18 -> Signal Conversion17/1  "<RoadCurvatureFar>"
  Signal Conversion17/1 -> Terminator17/1  "EHRV2_RoadCurvatureFar"
  Signal Conversion16/1 -> Terminator16/1  "EHRV2_RoadCurvature"
  Bus Selector/17 -> Signal Conversion16/1  "<RoadCurvature>"
  In3/1 -> Bus Creator2/3
  In4/1 -> Bus Creator2/4
  Bus Selector/28 -> Signal Conversion19/1  "<IFCHUTInterface>"
  Signal Conversion19/1 -> Terminator19/1  "EHRV2_IFCHUTInterface"
  Signal Conversion20/1 -> Terminator20/1  "EHRV2_MapDataValid"
  Bus Selector/29 -> Signal Conversion20/1  "<MapDataValid>"

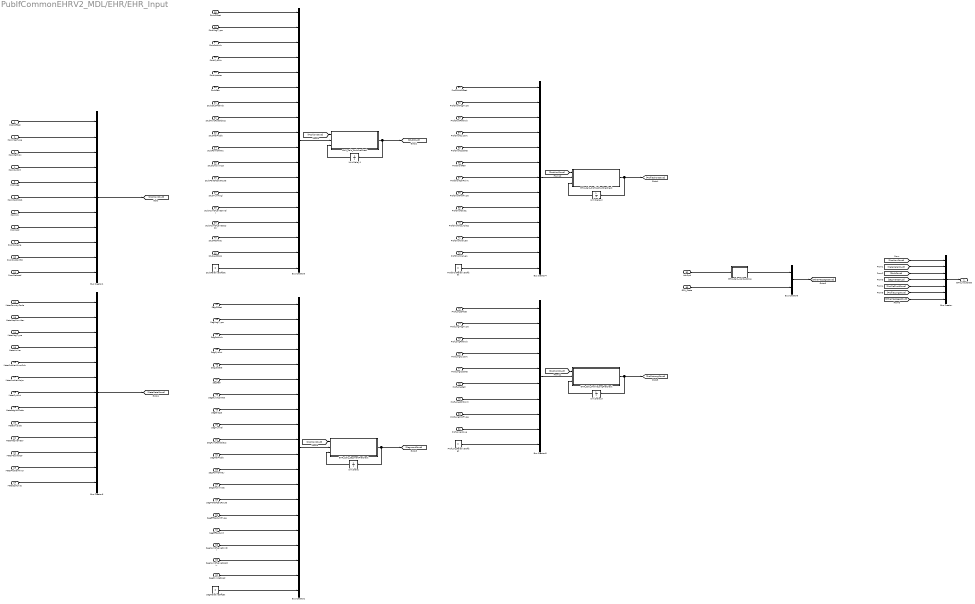
== system PubIfCommonEHRV2_MDL/EHR/EHR_Input ==
  PosnOffset : Inport
  PosnMsgType : Inport  Port=2
  PosnPathIdx : Inport  Port=3
  PosnCycCnt : Inport  Port=4
  PosnAge : Inport  Port=5
  PosnPosProbb : Inport  Port=6
  PosnIdx : Inport  Port=7
  PosnSpd : Inport  Port=8
  PosnCurLane : Inport  Port=9
  PosnPosConfdc : Inport  Port=10
  PosnRehead : Inport  Port=11
  MetaCountryCode : Inport  Port=12
  MetaMapProvider : Inport  Port=13
  MetaMsgType : Inport  Port=14
  MetaHwVer : Inport  Port=15
  MetaProtVerMinorSub : Inport  Port=16
  MetaProtVerMajor : Inport  Port=17
  MetaCycCnt : Inport  Port=18
  MetaRegionCode : Inport  Port=19
  MetaDrvSide : Inport  Port=20
  MetaMapVerYear : Inport  Port=21
  MetaMapVerQtr : Inport  Port=22
  MetaProtVerMinor : Inport  Port=23
  MetaSpdUnits : Inport  Port=24
  StubOffset : Inport  Port=25
  StubMsgType : Inport  Port=26
  StubPathIdx : Inport  Port=27
  StubCycCnt : Inport  Port=28
  StubUpdate : Inport  Port=29
  StubRetr : Inport  Port=30
  StubStubPathIdx : Inport  Port=31
  StubFuncRoadClass : Inport  Port=32
  StubRelProbb : Inport  Port=33
  StubFormOfWay : Inport  Port=34
  StubCmplxInsct : Inport  Port=35
  StubPartOfCalcRoute : Inport  Port=36
  StubTurnAngl : Inport  Port=37
  StubNumOfLaneDrvDir : Inport  Port=38
  StubNumOfLaneOppDir : Inport  Port=39
  StubRtOfWay : Inport  Port=40
  StubLastStub : Inport  Port=41
  SegOffset : Inport  Port=42
  SegMsgType : Inport  Port=43
  SegPathIdx : Inport  Port=44
  SegCycCnt : Inport  Port=45
  SegUpdate : Inport  Port=46
  SegRetr : Inport  Port=47
  SegBuildUpArea : Inport  Port=48
  SegBridge : Inport  Port=49
  SegTunnel : Inport  Port=50
  SegFuncRoadClass : Inport  Port=51
  SegRelProbb : Inport  Port=52
  SegFormOfWay : Inport  Port=53
  SegCmplxInsct : Inport  Port=54
  SegPartOfCalcRoute : Inport  Port=55
  SegEffSpdLmtType : Inport  Port=56
  SegEffSpdLmt : Inport  Port=57
  SegNumOfLaneDrvDir : Inport  Port=58
  SegNumOfLaneOppDir : Inport  Port=59
  SegDivideRoad : Inport  Port=60
  ProfShortOffset : Inport  Port=61
  ProfShortMsgType : Inport  Port=62
  ProfShortPathIdx : Inport  Port=63
  ProfShortCycCnt : Inport  Port=64
  ProfShortUpdate : Inport  Port=65
  ProfShortRetr : Inport  Port=66
  ProfShortCtrlPoint : Inport  Port=67
  ProfShortProfType : Inport  Port=68
  ProfShortDist1 : Inport  Port=69
  ProfShortAccurClass : Inport  Port=70
  ProfShortValue0 : Inport  Port=71
  ProfShortValue1 : Inport  Port=72
  ProfLongOffset : Inport  Port=73
  ProfLongMsgType : Inport  Port=74
  ProfLongPathIdx : Inport  Port=75
  ProfLongCycCnt : Inport  Port=76
  ProfLongUpdate : Inport  Port=77
  ProfLongRetr : Inport  Port=78
  ProfLongCtrlPoint : Inport  Port=79
  ProfLongProfType : Inport  Port=80
  ProfLongValue : Inport  Port=81
  VehSpd : Inport  Port=82
  ECU_State : Inport  Port=83
  Bus Creator : BusCreator  Inputs=7
  Bus Creator1 : BusCreator  Inputs=11  OutDataTypeStr=Bus: PositionStruct  NonVirtualBus=on
  Bus Creator2 : BusCreator  Inputs=20  OutDataTypeStr=Bus: SegmentStruct  NonVirtualBus=on
  Bus Creator3 : BusCreator  Inputs=18  OutDataTypeStr=Bus: StubStruct  NonVirtualBus=on
  Bus Creator4 : BusCreator  Inputs=13  OutDataTypeStr=Bus: ProfileShortStruct  NonVirtualBus=on
  Bus Creator5 : BusCreator  Inputs=10  OutDataTypeStr=Bus: ProfileLongStruct  NonVirtualBus=on
  Bus Creator6 : BusCreator  Inputs=13  OutDataTypeStr=Bus: MetaDataStruct  NonVirtualBus=on
  Bus Creator8 : BusCreator  Inputs=2
  EHR_Calc_ProfileLongPreCheck : MATLAB Function  TreatAsAtomicUnit=on
  EHR_Calc_ProfileShortPreCheck : MATLAB Function  TreatAsAtomicUnit=on
  EHR_Calc_SegmentPreCheck : MATLAB Function  TreatAsAtomicUnit=on
  EHR_Calc_StubPreCheck : MATLAB Function  TreatAsAtomicUnit=on
  EHR_Calc_VehSpdDisp : MATLAB Function  TreatAsAtomicUnit=on
  ProfLongRelativeOffset : Constant  Value=0  OutDataTypeStr=int16
  ProfShortRelativeOffset : Constant  Value=0  OutDataTypeStr=int16
  SegRelativeOffset : Constant  Value=0  OutDataTypeStr=int16
  StubRelativeOffset : Constant  Value=0  OutDataTypeStr=int16
  Unit Delay{,1..3} (4 alike) : UnitDelay  SampleTime=-1  HasFrameUpgradeWarning=on
  EHR_InputData : Outport
  wires:
  Bus Creator6/1 -> [MetaDataStruct]
  Bus Creator1/1 -> [PositionStruct]
  Bus Creator8/1 -> [OtherMessageStruct]
  [PositionStruct] -> Bus Creator/1  "PositionStruct"
  [MetaDataStruct] -> Bus Creator/2  "MetaDataStruct"
  [OtherMessageStruct] -> Bus Creator/7  "OtherMessageStruct"
  [ProfileLongStruct] -> Bus Creator/6  "ProfileLongStruct"
  [ProfileShortStruct] -> Bus Creator/5  "ProfileShortStruct"
  [SegmentStruct] -> Bus Creator/4  "SegmentStruct"
  [StubStruct] -> Bus Creator/3  "StubStruct"
  Bus Creator/1 -> EHR_InputData/1
  StubRelativeOffset/1 -> Bus Creator3/18  "StubRelativeOffset"
  SegRelativeOffset/1 -> Bus Creator2/20  "SegRelativeOffset"
  EHR_Calc_SegmentPreCheck/1(SegmentStructOut) -> [SegmentStruct], Unit Delay/1
  Bus Creator2/1 -> EHR_Calc_SegmentPreCheck/2(SegmentStructIn)
  [PositionStruct] -> EHR_Calc_SegmentPreCheck/1(PositionStructIn)
  Unit Delay/1 -> EHR_Calc_SegmentPreCheck/3(SegmentStructOutK1)
  Bus Creator3/1 -> EHR_Calc_StubPreCheck/2(StubStructIn)
  [PositionStruct] -> EHR_Calc_StubPreCheck/1(PositionStructIn)
  EHR_Calc_StubPreCheck/1(StubStructOut) -> [StubStruct], Unit Delay1/1
  Unit Delay1/1 -> EHR_Calc_StubPreCheck/3(StubStructOutK1)
  ProfShortRelativeOffset/1 -> Bus Creator4/13  "ProfShortRelativeOffset"
  EHR_Calc_ProfileShortPreCheck/1(ProfileShortStructOut) -> [ProfileShortStruct], Unit Delay2/1
  [PositionStruct] -> EHR_Calc_ProfileShortPreCheck/1(PositionStructIn)
  Bus Creator4/1 -> EHR_Calc_ProfileShortPreCheck/2(ProfileShortStructIn)
  Unit Delay2/1 -> EHR_Calc_ProfileShortPreCheck/3(ProfileShortStructOutK1)
  ProfLongRelativeOffset/1 -> Bus Creator5/10  "ProfLongRelativeOffset"
  [PositionStruct] -> EHR_Calc_ProfileLongPreCheck/1(PositionStructIn)
  EHR_Calc_ProfileLongPreCheck/1(ProfileLongStructOut) -> [ProfileLongStruct], Unit Delay3/1
  Bus Creator5/1 -> EHR_Calc_ProfileLongPreCheck/2(ProfileLongStructIn)
  Unit Delay3/1 -> EHR_Calc_ProfileLongPreCheck/3(ProfileLongStructOutK1)
  EHR_Calc_VehSpdDisp/1(VehSpdDisp) -> Bus Creator8/1  "VehSpdDisp"
  PosnOffset/1 -> Bus Creator1/1  "PosnOffset"
  PosnMsgType/1 -> Bus Creator1/2  "PosnMsgType"
  PosnPathIdx/1 -> Bus Creator1/3  "PosnPathIdx"
  PosnAge/1 -> Bus Creator1/5  "PosnAge"
  PosnCycCnt/1 -> Bus Creator1/4  "PosnCycCnt"
  PosnPosProbb/1 -> Bus Creator1/6  "PosnPosProbb"
  PosnSpd/1 -> Bus Creator1/8  "PosnSpd"
  PosnCurLane/1 -> Bus Creator1/9  "PosnCurLane"
  PosnIdx/1 -> Bus Creator1/7  "PosnIdx"
  PosnPosConfdc/1 -> Bus Creator1/10  "PosnPosConfdc"
  PosnRehead/1 -> Bus Creator1/11  "PosnRehead"
  MetaCountryCode/1 -> Bus Creator6/1  "MetaCountryCode"
  MetaMapProvider/1 -> Bus Creator6/2  "MetaMapProvider"
  MetaMsgType/1 -> Bus Creator6/3  "MetaMsgType"
  MetaHwVer/1 -> Bus Creator6/4  "MetaHwVer"
  MetaProtVerMinorSub/1 -> Bus Creator6/5  "MetaProtVerMinorSub"
  MetaProtVerMajor/1 -> Bus Creator6/6  "MetaProtVerMajor"
  MetaRegionCode/1 -> Bus Creator6/8  "MetaRegionCode"
  MetaCycCnt/1 -> Bus Creator6/7  "MetaCycCnt"
  MetaDrvSide/1 -> Bus Creator6/9  "MetaDrvSide"
  MetaMapVerYear/1 -> Bus Creator6/10  "MetaMapVerYear"
  MetaMapVerQtr/1 -> Bus Creator6/11  "MetaMapVerQtr"
  MetaProtVerMinor/1 -> Bus Creator6/12  "MetaProtVerMinor"
  MetaSpdUnits/1 -> Bus Creator6/13  "MetaSpdUnits"
  StubOffset/1 -> Bus Creator3/1  "StubOffset"
  StubMsgType/1 -> Bus Creator3/2  "StubMsgType"
  StubPathIdx/1 -> Bus Creator3/3  "StubPathIdx"
  StubCycCnt/1 -> Bus Creator3/4  "StubCycCnt"
  StubRelProbb/1 -> Bus Creator3/9  "StubRelProbb"
  StubStubPathIdx/1 -> Bus Creator3/7  "StubStubPathIdx"
  StubFuncRoadClass/1 -> Bus Creator3/8  "StubFuncRoadClass"
  StubFormOfWay/1 -> Bus Creator3/10  "StubFormOfWay"
  StubCmplxInsct/1 -> Bus Creator3/11  "StubCmplxInsct"
  StubPartOfCalcRoute/1 -> Bus Creator3/12  "StubPartOfCalcRoute"
  StubNumOfLaneOppDir/1 -> Bus Creator3/15  "StubNumOfLaneOppDir"
  StubTurnAngl/1 -> Bus Creator3/13  "StubTurnAngl"
  StubNumOfLaneDrvDir/1 -> Bus Creator3/14  "StubNumOfLaneDrvDir"
  StubRtOfWay/1 -> Bus Creator3/16  "StubRtOfWay"
  SegOffset/1 -> Bus Creator2/1  "SegOffset"
  SegMsgType/1 -> Bus Creator2/2  "SegMsgType"
  SegPathIdx/1 -> Bus Creator2/3  "SegPathIdx"
  SegCycCnt/1 -> Bus Creator2/4  "SegCycCnt"
  SegBuildUpArea/1 -> Bus Creator2/7  "SegBuildUpArea"
  SegFormOfWay/1 -> Bus Creator2/12  "SegFormOfWay"
  SegFuncRoadClass/1 -> Bus Creator2/10  "SegFuncRoadClass"
  SegRelProbb/1 -> Bus Creator2/11  "SegRelProbb"
  SegTunnel/1 -> Bus Creator2/9  "SegTunnel"
  SegBridge/1 -> Bus Creator2/8  "SegBridge"
  SegCmplxInsct/1 -> Bus Creator2/13  "SegCmplxInsct"
  SegEffSpdLmtType/1 -> Bus Creator2/15  "SegEffSpdLmtType"
  SegPartOfCalcRoute/1 -> Bus Creator2/14  "SegPartOfCalcRoute"
  SegEffSpdLmt/1 -> Bus Creator2/16  "SegEffSpdLmt"
  SegNumOfLaneOppDir/1 -> Bus Creator2/18  "SegNumOfLaneOppDir"
  SegNumOfLaneDrvDir/1 -> Bus Creator2/17  "SegNumOfLaneDrvDir"
  SegDivideRoad/1 -> Bus Creator2/19  "SegDivideRoad"
  ProfShortOffset/1 -> Bus Creator4/1  "ProfShortOffset"
  ProfShortMsgType/1 -> Bus Creator4/2  "ProfShortMsgType"
  ProfShortPathIdx/1 -> Bus Creator4/3  "ProfShortPathIdx"
  ProfShortCycCnt/1 -> Bus Creator4/4  "ProfShortCycCnt"
  ProfShortProfType/1 -> Bus Creator4/8  "ProfShortProfType"
  ProfShortDist1/1 -> Bus Creator4/9  "ProfShortDist1"
  ProfShortValue0/1 -> Bus Creator4/11  "ProfShortValue0"
  ProfShortValue1/1 -> Bus Creator4/12  "ProfShortValue1"
  ProfShortAccurClass/1 -> Bus Creator4/10  "ProfShortAccurClass"
  ProfLongOffset/1 -> Bus Creator5/1  "ProfLongOffset"
  ProfLongMsgType/1 -> Bus Creator5/2  "ProfLongMsgType"
  ProfLongPathIdx/1 -> Bus Creator5/3  "ProfLongPathIdx"
  ProfLongCycCnt/1 -> Bus Creator5/4  "ProfLongCycCnt"
  ProfLongProfType/1 -> Bus Creator5/8  "ProfLongProfType"
  ProfLongValue/1 -> Bus Creator5/9  "ProfLongValue"
  VehSpd/1 -> EHR_Calc_VehSpdDisp/1(VehSpd)  "VehSpd"
  ECU_State/1 -> Bus Creator8/2  "ECU_State"
  StubUpdate/1 -> Bus Creator3/5  "StubUpdate"
  StubRetr/1 -> Bus Creator3/6  "StubRetr"
  StubLastStub/1 -> Bus Creator3/17  "StubLastStub"
  SegUpdate/1 -> Bus Creator2/5  "SegUpdate"
  SegRetr/1 -> Bus Creator2/6  "SegRetr"
  ProfShortUpdate/1 -> Bus Creator4/5  "ProfShortUpdate"
  ProfShortRetr/1 -> Bus Creator4/6  "ProfShortRetr"
  ProfShortCtrlPoint/1 -> Bus Creator4/7  "ProfShortCtrlPoint"
  ProfLongUpdate/1 -> Bus Creator5/5  "ProfLongUpdate"
  ProfLongRetr/1 -> Bus Creator5/6  "ProfLongRetr"
  ProfLongCtrlPoint/1 -> Bus Creator5/7  "ProfLongCtrlPoint"
